simulink model "lab6t1"  (Simulink 9.3)
settings: Solver=ode45  StartTime=0.0  StopTime=10.0  RelTol=1e-3  EnableMultiTasking=on
settings Model: Creator=Muhammad Ali khan  LastModifiedBy=Muhammad Ali khan
settings DataIOCC: LimitDataPoints=on
settings OptimizationCC: ExpressionDepthLimit=2147483647
settings DebuggingCC: SolverPrmCheckMsg=warning  StateNameClashWarn=warning
settings GRTTargetCC: GeneratePreprocessorConditionals=Disable all

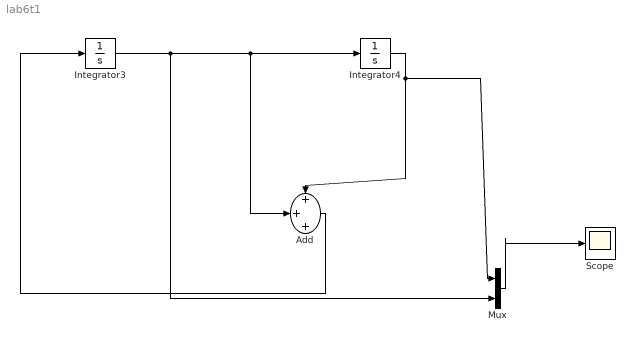
== system lab6t1 ==
  Add : Sum  Inputs=+++
  Integrator3 : Integrator  InitialCondition=2
  Integrator4 : Integrator  InitialCondition=1
  Mux : Mux  Inputs=2
  Scope : Scope
  wires:
  Integrator3/1 -> Mux/2, Integrator4/1, Add/2
  Integrator4/1 -> Mux/1, Add/1
  Mux/1 -> Scope/1
  Add/1 -> Integrator3/1
